simulink model "emissionversion"  (R2024b)
settings: Solver=FixedStepAuto  StartTime=0.0  StopTime=200  RelTol=1e-3  EnableMultiTasking=on
PreLoadFcn:
  | try, eval([bdroot '_setup']); catch, eval('model_setup', ''); end
InitFcn:
  | try, eval([bdroot '_setup']); catch, eval('model_setup', ''); end
model workspace (MAT data in the model file):
  PID_rpm = [1000 2000 3000 4000]
undefined symbols (not defined in the file): ECU555, motohawk_build_version, motohawk_get_target_image, motohawk_target_type, motohawk_trunc_name, motohawk_vardec_path
libraries: MotoHawk_lib x118, motohawk_annotations_lib x23, dspstat3 x13, drivingcycle_lib x1, motohawk_examples_lib x1, MotoHawk_Protocols_lib x1
(part 4 of 5)

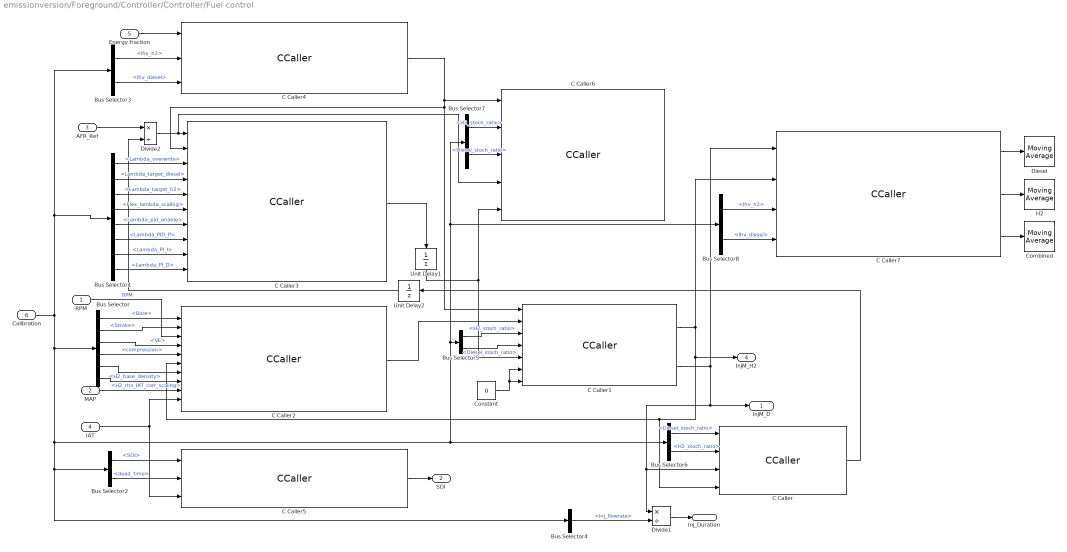
== system emissionversion/Foreground/Controller/Controller/Fuel control ==
  RPM : Inport
  MAP : Inport  Port=2
  AFR_Ref : Inport  Port=3
  IAT : Inport  Port=4
  Energy fraction : Inport  Port=5
  Calibration : Inport  Port=6
  Bus Selector : BusSelector  OutputSignals=signal1.Bore,signal1.Stroke,signal1.VE,signal1.compression,signal1.H2_base_density,signal1.H2_rho_IAT_corr_scaling
  Bus Selector1 : BusSelector  OutputSignals=signal1.Lambda_overwrite,signal1.Lambda_target_diesel,signal1.Lambda_target_h2,signal1.Flex_lambda_scaling,signal1.Lambda_pid_enable,signal1.Lambda_PID_P,signal1.Lambda_PI_I,signal1.Lambda_PI_D
  Bus Selector2 : BusSelector  OutputSignals=signal1.SOI,signal1.dead_time
  Bus Selector3 : BusSelector  OutputSignals=signal1.lhv_h2,signal1.lhv_diesel
  Bus Selector4 : BusSelector  OutputSignals=signal1.Inj_flowrate
  Bus Selector5 : BusSelector  OutputSignals=signal1.H2_stoch_ratio,signal1.Diesel_stoch_ratio
  Bus Selector6 : BusSelector  OutputSignals=signal1.Diesel_stoch_ratio,signal1.H2_stoch_ratio
  Bus Selector7 : BusSelector  OutputSignals=signal1.H2_stoch_ratio,signal1.Diesel_stoch_ratio
  Bus Selector8 : BusSelector  OutputSignals=signal1.lhv_h2,signal1.lhv_diesel
  C Caller : CCaller  FunctionName=calculateCombinedAFR  PortSpecificationStruct="%)30     .    * D   8    (     @         %    \"     4    !     0         %  0 \"0    $    _    07)G3F%M90  4&]R=$YA;64 4V-O<&4     26YD97@     5'EP90      4VEZ90      27-';&]B86P   X    P    !@    @    $          4    (     0    ,    !         !   P!O=70 #@   #     &    \"     0         !0    @    !     P    $         $  # &]U=  .    .     8    (    !          %    \"     $    &     0         0   ...(+2774 chars)"
  C Caller1 : CCaller  FunctionName=Injection_amounts  PortSpecificationStruct="%)30     .    .!    8    (     @         %    \"     D    !     0         %  0 \"0    $    _    07)G3F%M90  4&]R=$YA;64 4V-O<&4     26YD97@     5'EP90      4VEZ90      27-';&]B86P   X   !     !@    @    $          4    (     0    T    !         !     -    ;6%S<U]F<F%C=&EO;@    X   !     !@    @    $          4    (     0    T    !         !     -    ;6%S<U]F<F%C=&EO;@    X    X    !@    @    $     ...(+5220 chars)"
  C Caller2 : CCaller  FunctionName=airMassCalc  PortSpecificationStruct="%)30     .    6!,   8    (     @         %    \"     L    !     0         %  0 \"0    $    _    07)G3F%M90  4&]R=$YA;64 4V-O<&4     26YD97@     5'EP90      4VEZ90      27-';&]B86P   X    P    !@    @    $          4    (     0    0    !         !  ! !B;W)E#@   #     &    \"     0         !0    @    !    !     $         $  $ &)O<F4.    .     8    (    !          %    \"     $    %     0         0   ...(+6292 chars)"
  C Caller3 : CCaller  FunctionName=LambdaControl  PortSpecificationStruct="%)30     .    N!,   8    (     @         %    \"     L    !     0         %  0 \"0    $    _    07)G3F%M90  4&]R=$YA;64 4V-O<&4     26YD97@     5'EP90      4VEZ90      27-';&]B86P   X   !     !@    @    $          4    (     0   !     !         !     0    ;&%M8F1A7W)E9F5R96YC90X   !     !@    @    $          4    (     0   !     !         !     0    ;&%M8F1A7W)E9F5R96YC90X    X    !@    @    $     ...(+6421 chars)"
  C Caller4 : CCaller  FunctionName=mass_fraction_calc  PortSpecificationStruct="%)30     .    J <   8    (     @         %    \"     0    !     0         %  0 \"0    $    _    07)G3F%M90  4&]R=$YA;64 4V-O<&4     26YD97@     5'EP90      4VEZ90      27-';&]B86P   X   !     !@    @    $          4    (     0    \\    !         !     /    96YE<F=Y7V9R86-T:6]N  X   !     !@    @    $          4    (     0    \\    !         !     /    96YE<F=Y7V9R86-T:6]N  X    X    !@    @    $   ...(+2256 chars)"
  C Caller5 : CCaller  FunctionName=start_of_injection  PortSpecificationStruct="%)30     .    * <   8    (     @         %    \"     0    !     0         %  0 \"0    $    _    07)G3F%M90  4&]R=$YA;64 4V-O<&4     26YD97@     5'EP90      4VEZ90      27-';&]B86P   X    X    !@    @    $          4    (     0    @    !         !     (    <V]I7V)A<V4.    .     8    (    !          %    \"     $    (     0         0    \"    '-O:5]B87-E#@   #@    &    \"     0         !0    @    !  ...(+2083 chars)"
  C Caller6 : CCaller  FunctionName=s_fuel_trim_calc  PortSpecificationStruct="%)30     .    R P   8    (     @         %    \"     <    !     0         %  0 \"0    $    _    07)G3F%M90  4&]R=$YA;64 4V-O<&4     26YD97@     5'EP90      4VEZ90      27-';&]B86P   X   !     !@    @    $          4    (     0    T    !         !     -    ;6%S<U]F<F%C=&EO;@    X   !     !@    @    $          4    (     0    T    !         !     -    ;6%S<U]F<F%C=&EO;@    X    X    !@    @    $     ...(+4021 chars)"
  C Caller7 : CCaller  FunctionName=energy_monitor  PortSpecificationStruct="%)30     .    R P   8    (     @         %    \"     <    !     0         %  0 \"0    $    _    07)G3F%M90  4&]R=$YA;64 4V-O<&4     26YD97@     5'EP90      4VEZ90      27-';&]B86P   X    X    !@    @    $          4    (     0    <    !         !     '    :6YJ7VU?9  .    .     8    (    !          %    \"     $    '     0         0    !P   &EN:E]M7V0 #@   #@    &    \"     0         !0    @    !   ...(+4024 chars)"
  Combined : dspstat3/Moving Average  Method=Sliding window  ForgettingFactorPort=off  SpecifyWindowLength=on  WindowLength=200  OverlapLength=199  AllowArbitraryInputLength=off  ForgettingFactor=0.9  SimulateUsing=Interpreted execution
  Constant : Constant  Value=0
  Diesel : dspstat3/Moving Average  Method=Sliding window  ForgettingFactorPort=off  SpecifyWindowLength=on  WindowLength=200  OverlapLength=199  AllowArbitraryInputLength=off  ForgettingFactor=0.9  SimulateUsing=Interpreted execution
  Divide1 : Product  Inputs=*/
  Divide2 : Product  Inputs=*/
  H2 : dspstat3/Moving Average  Method=Sliding window  ForgettingFactorPort=off  SpecifyWindowLength=on  WindowLength=200  OverlapLength=199  AllowArbitraryInputLength=off  ForgettingFactor=0.9  SimulateUsing=Interpreted execution
  Unit Delay1 : UnitDelay  SampleTime=-1  HasFrameUpgradeWarning=on
  Unit Delay2 : UnitDelay  SampleTime=-1  HasFrameUpgradeWarning=on
  InjM_D : Outport
  SOI : Outport  Port=2
  Inj_Duration : Outport  Port=3
  InjM_H2 : Outport  Port=4
  wires:
  Energy fraction/1 -> C Caller4/1
  AFR_Ref/1 -> Divide2/1
  Calibration/1 -> Bus Selector6/1, Bus Selector8/1, Bus Selector7/1, Bus Selector5/1, Bus Selector4/1, Bus Selector2/1, Bus Selector/1, Bus Selector1/1, Bus Selector3/1
  RPM/1 -> C Caller2/3  "RPM"
  C Caller5/1 -> SOI/1
  MAP/1 -> C Caller2/9
  Bus Selector/1 -> C Caller2/1  "<Bore>"
  Bus Selector/2 -> C Caller2/2  "<Stroke>"
  Bus Selector/3 -> C Caller2/4  "<VE>"
  Bus Selector/4 -> C Caller2/5  "<compression>"
  Bus Selector/5 -> C Caller2/7  "<H2_base_density>"
  Bus Selector/6 -> C Caller2/8  "<H2_rho_IAT_corr_scaling>"
  IAT/1 -> C Caller5/3, C Caller2/10
  C Caller4/1 -> C Caller1/1, C Caller3/2, C Caller6/1
  C Caller2/1 -> C Caller1/2
  C Caller1/1 -> C Caller7/2, InjM_H2/1, C Caller2/6, C Caller/4
  Divide1/1 -> Inj_Duration/1
  C Caller/1 -> Unit Delay2/1
  C Caller1/2 -> C Caller7/1, Divide1/1, C Caller/3, InjM_D/1
  Divide2/1 -> C Caller6/4, C Caller3/1
  C Caller3/1 -> Unit Delay1/1
  Bus Selector1/1 -> C Caller3/3  "<Lambda_overwrite>"
  Bus Selector1/2 -> C Caller3/4  "<Lambda_target_diesel>"
  Bus Selector1/3 -> C Caller3/5  "<Lambda_target_h2>"
  Bus Selector1/4 -> C Caller3/6  "<Flex_lambda_scaling>"
  Bus Selector1/5 -> C Caller3/7  "<Lambda_pid_enable>"
  Bus Selector1/6 -> C Caller3/8  "<Lambda_PID_P>"
  Bus Selector1/7 -> C Caller3/9  "<Lambda_PI_I>"
  Bus Selector1/8 -> C Caller3/10  "<Lambda_PI_D>"
  Bus Selector2/1 -> C Caller5/1  "<SOI>"
  Bus Selector2/2 -> C Caller5/2  "<dead_time>"
  Bus Selector3/2 -> C Caller4/3  "<lhv_diesel>"
  Bus Selector3/1 -> C Caller4/2  "<lhv_h2>"
  Unit Delay1/1 -> C Caller1/5, C Caller6/5
  Bus Selector4/1 -> Divide1/2  "<Inj_flowrate>"
  Bus Selector5/1 -> C Caller1/3  "<H2_stoch_ratio>"
  Bus Selector5/2 -> C Caller1/4  "<Diesel_stoch_ratio>"
  Bus Selector6/1 -> C Caller/1  "<Diesel_stoch_ratio>"
  Bus Selector6/2 -> C Caller/2  "<H2_stoch_ratio>"
  Bus Selector7/1 -> C Caller6/2  "<H2_stoch_ratio>"
  Bus Selector7/2 -> C Caller6/3  "<Diesel_stoch_ratio>"
  Unit Delay2/1 -> Divide2/2
  Bus Selector8/2 -> C Caller7/4  "<lhv_diesel>"
  Bus Selector8/1 -> C Caller7/3  "<lhv_h2>"
  C Caller7/3 -> Combined/1
  C Caller7/2 -> H2/1
  C Caller7/1 -> Diesel/1
  Constant/1 -> C Caller1/6, C Caller1/7
